simulink model "simModel"  (R2020a)
settings: Solver=VariableStepAuto  StartTime=0.0  StopTime=1  RelTol=1e-3
libraries: environment x1, plant x1, controller x1
settings Model: Creator=Ayaz  LastModifiedBy=Ayaz

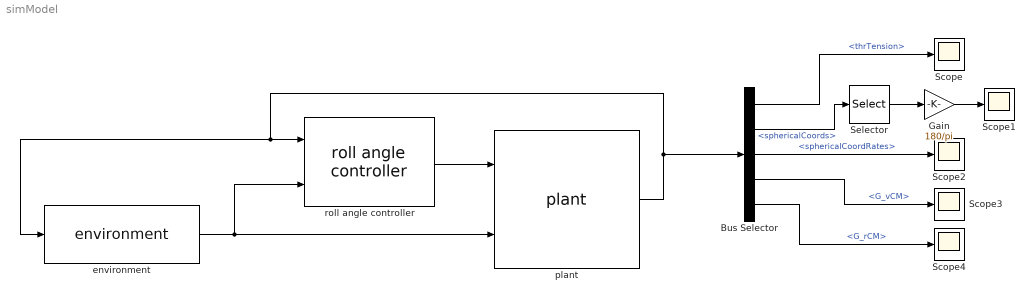
== system simModel ==
  Bus Selector : BusSelector  OutputSignals=thrTension,sphericalCoords,sphericalCoordRates,G_vCM,G_rCM
  Gain : Gain  Gain=180/pi
  Scope{,1..4} (5 alike) : Scope
  Selector : Selector  InputPortWidth=3  IndexOptions=Index vector (dialog)  Indices=[1 2]  OutputSizes=1
  environment : environment/environment  LabelModeActiveChoice=v1  flowTypeVar=Constant flow  flowSpeed=flowSpeed  Parameter3=0
  plant : plant/plant  AoA=AoA  init_radius=init_R  init_azim=init_azim  init_elev=init_elev  init_dAzim=init_azimRate  init_dElev=init_elevRate  gravEnable=on  fluidEnable=on  mass=kiteMass  refArea=refArea  aeroCent=aeroCent  AoA_vals=AoA_vals  CL_vals=CL_vals  CD_vals=CD_vals  flowDensity=rho  gravAccel=gravAccl
  roll angle controller : controller/roll angle controller  SystemSampleTime=-1  Latency=0  AutoFrameSizeCalculation=off
  wires:
  roll angle controller/1 -> plant/1
  environment/1 -> roll angle controller/2, plant/2
  plant/1 -> Bus Selector/1, environment/1, roll angle controller/1
  Bus Selector/1 -> Scope/1  "<thrTension>"
  Bus Selector/2 -> Selector/1  "<sphericalCoords>"
  Bus Selector/3 -> Scope2/1  "<sphericalCoordRates>"
  Selector/1 -> Gain/1
  Bus Selector/4 -> Scope3/1  "<G_vCM>"
  Bus Selector/5 -> Scope4/1  "<G_rCM>"
  Gain/1 -> Scope1/1
